simulink model "cube0_mpcpd"  (R2022b)
settings: Solver=VariableStepAuto  StartTime=0.0  StopTime=400  RelTol=1e-3  AbsTol=1e-3
undefined symbols (not defined in the file or in its folder): Angle, Axis
libraries: robotcorelib x2
settings Model: Creator=Abhijit  LastModifiedBy=abhij
settings SolverCC: AutoScaleAbsTol=off  AlgebraicLoopSolver=TrustRegion  MaxZcPerStep=1
settings DebuggingCC: UnconnectedInputMsg=warning  UnconnectedOutputMsg=warning  UnconnectedLineMsg=warning  SymbolicDimsDataTypeCodeGenerationDiagnostic=none  SFMachineParentedDataDiag=warning
settings ModelReferenceCC: EnableRefExpFcnMdlSchedulingChecks=on
settings SFSimCC: CustomCodeUndefinedFunction=UseInterfaceOnly
settings RTWCC: DLArmComputeVersion=19.05
settings SimscapeCC: SimscapeLogType=all  SimscapeLogSimulationStatistics=on  SimscapeLogDataHistory=10000

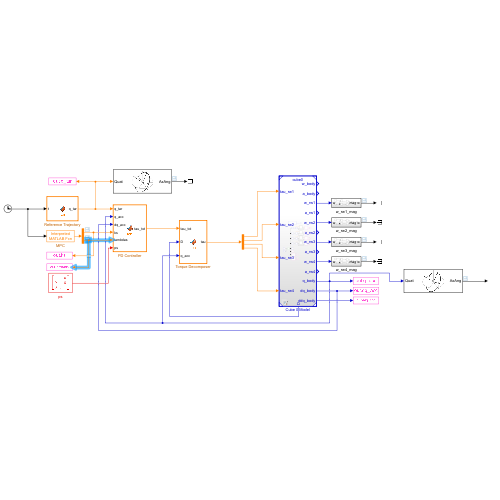
[thumbnail: Simulink's stored preview of the top-level diagram]
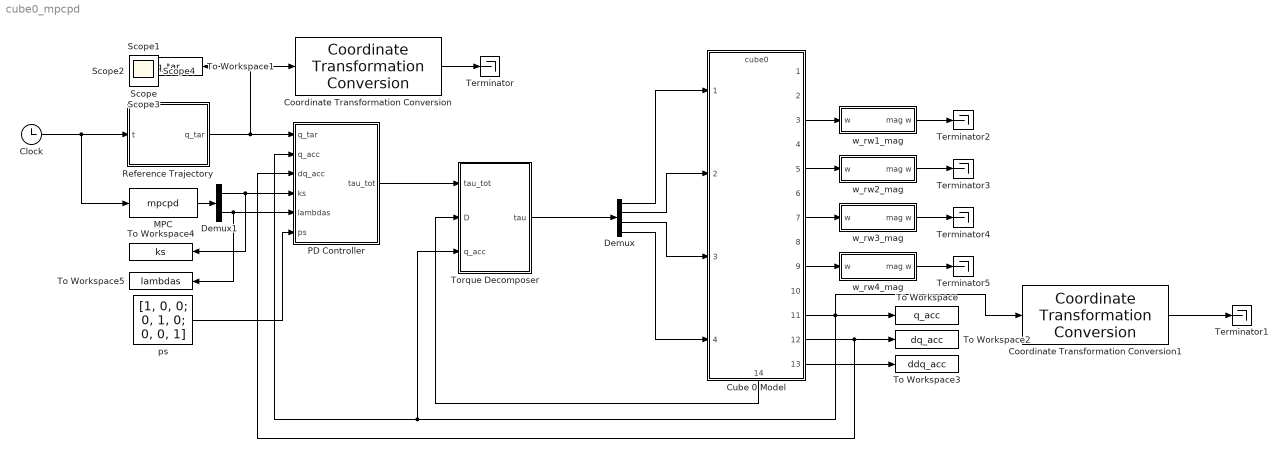
== system cube0_mpcpd ==
  Clock : Clock
  Coordinate Transformation Conversion : robotcorelib/Coordinate Transformation Conversion  InputRepresentation=Quaternion  InputEulerSequence=ZYX  ShowTrVecInputPort=on  OutputRepresentation=Axis-Angle  OutputEulerSequence=ZYX  ShowTrVecOutputPort=on  SimulateUsing=Interpreted execution
      settings: LibrarySourceBlock=navlib/Utilities/Coordinate Transformation Conversion
  Coordinate Transformation Conversion1 : robotcorelib/Coordinate Transformation Conversion  InputRepresentation=Quaternion  InputEulerSequence=ZYX  ShowTrVecInputPort=on  OutputRepresentation=Axis-Angle  OutputEulerSequence=ZYX  ShowTrVecOutputPort=on  SimulateUsing=Interpreted execution
      settings: LibrarySourceBlock=navlib/Utilities/Coordinate Transformation Conversion
  Cube 0 Model : ModelReference  ModelNameDialog=cube0.slx  SimulationMode=Normal  ModelReferenceVersion=1.24
      settings: PortSchema="{\"entries\":[{\"content\":{\"sides\":[{\"content\":{\"connectorIds\":[\"In1\",\"In2\",\"In3\",\"In4\"]},\"type\":\"ConnectorPlacement.EquallySpacedRectSide\",\"uuid\":\"36a9c944-f213-4c4e-b6f2-fa7d728627b0\"},{\"content\":{\"connectorIds\":[\"Out1\",\"Out2\",\"Out3\",\"Out4\",\"Out5\",\"Out6\",\"Out7\",\"Out8\",\"Out9\",\"Out10\",\"Out11\",\"Out12\",\"Out13\"],\"side\":\"RIGHT\"},\"type\":\"ConnectorPlacement.EquallySpacedRectSide\",\"uuid\":\"ad793041-f32f-405f-9966-9455be290c1c\"},{\"content\":{\"connectorIds\":[],\"side\":\"TOP\"},\"type\":\"ConnectorPlacement.EquallySpacedRectSide\",\"uuid\":\"a8d37d27-2c3a-480b-9200-d310321df053\"},{\"content\":{\"connectorIds\":[\"Out14\"],\"side\":\"BOTTOM\"},\"type\":\"ConnectorPlacement.EquallySpacedRectSide\",\"uuid\":\"42546c36-6810-4b9b-bafe-a7a09e10a567\"}]},\"type\":\"ConnectorPlacement.EquallySpacedConnector\",\"uuid\":\"5842ca05-faf4-4c84-934b-15246120a6a0\"}],\"packageUris\":[\"http://schema.mathworks.com/mf0/Connector/R2020b\"],\"version\":\"1.0\"}"
  Demux : Demux
  Demux1 : Demux  Outputs=2
  MPC : MATLABFcn  MATLABFcn=mpcpd  OutputDimensions=6
  PD Controller : MATLAB Function  TreatAsAtomicUnit=on
  Reference Trajectory : MATLAB Function  TreatAsAtomicUnit=on
  Terminator{,1..5} (6 alike) : Terminator
  To Workspace : ToWorkspace  VariableName=q_acc  SaveFormat=Timeseries  SampleTime=-1
  To Workspace1 : ToWorkspace  VariableName=q_tar  SaveFormat=Timeseries  SampleTime=-1
  To Workspace2 : ToWorkspace  VariableName=dq_acc  SaveFormat=Timeseries  SampleTime=-1
  To Workspace3 : ToWorkspace  VariableName=ddq_acc  SaveFormat=Timeseries  SampleTime=-1
  To Workspace4 : ToWorkspace  VariableName=ks  SaveFormat=Timeseries  SampleTime=-1
  To Workspace5 : ToWorkspace  VariableName=lambdas  SaveFormat=Timeseries  SampleTime=-1
  Torque Decomposer : MATLAB Function  TreatAsAtomicUnit=on
  ps : Constant  Value=[1, 0, 0; 0, 1, 0; 0, 0, 1]
  w_rw1_mag : Subsystem
  w_rw2_mag : Subsystem
  w_rw3_mag : Subsystem
  w_rw4_mag : Subsystem
  Scope{,1..4} (5 alike) : Scope
  wires:
  Clock/1 -> MPC/1, Reference Trajectory/1(t)
  Demux1/2 -> PD Controller/5(lambdas), To Workspace5/1
  Demux1/1 -> PD Controller/4(ks), To Workspace4/1
  ps/1 -> PD Controller/6(ps)
  Reference Trajectory/1(q_tar) -> Coordinate Transformation Conversion/1, To Workspace1/1, PD Controller/1(q_tar)
  MPC/1 -> Demux1/1
  Coordinate Transformation Conversion/1 -> Terminator/1
  w_rw3_mag/1(mag w) -> Terminator4/1
  Cube 0 Model/5 -> w_rw2_mag/1(w)
  w_rw1_mag/1(mag w) -> Terminator2/1
  Cube 0 Model/12 -> PD Controller/3(dq_acc), To Workspace2/1
  Cube 0 Model/9 -> w_rw4_mag/1(w)
  Demux/2 -> Cube 0 Model/2
  Cube 0 Model/7 -> w_rw3_mag/1(w)
  Cube 0 Model/3 -> w_rw1_mag/1(w)
  w_rw4_mag/1(mag w) -> Terminator5/1
  Demux/3 -> Cube 0 Model/3
  Cube 0 Model/13 -> To Workspace3/1
  Demux/4 -> Cube 0 Model/4
  Demux/1 -> Cube 0 Model/1
  Coordinate Transformation Conversion1/1 -> Terminator1/1
  Cube 0 Model/14 -> Torque Decomposer/2(D)
  w_rw2_mag/1(mag w) -> Terminator3/1
  Cube 0 Model/11 -> To Workspace/1, Coordinate Transformation Conversion1/1, PD Controller/2(q_acc), Torque Decomposer/3(q_acc)
  Torque Decomposer/1(tau) -> Demux/1
  PD Controller/1(tau_tot) -> Torque Decomposer/1(tau_tot)

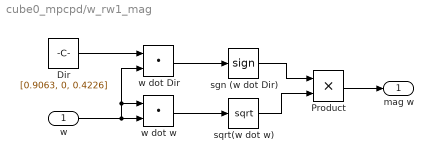
== system cube0_mpcpd/w_rw1_mag ==
  w : Inport
  Dir : Constant  Value=[0.9063, 0, 0.4226]
  Product : Product
  sgn (w dot Dir) : Signum
  sqrt(w dot w) : Sqrt
  w dot Dir : DotProduct  OutDataTypeStr=Inherit: Inherit via internal rule
  w dot w : DotProduct  OutDataTypeStr=Inherit: Inherit via internal rule
  mag w : Outport
  wires:
  w dot Dir/1 -> sgn (w dot Dir)/1
  w/1 -> w dot Dir/2, w dot w/1, w dot w/2
  w dot w/1 -> sqrt(w dot w)/1
  Product/1 -> mag w/1
  sqrt(w dot w)/1 -> Product/2
  Dir/1 -> w dot Dir/1
  sgn (w dot Dir)/1 -> Product/1

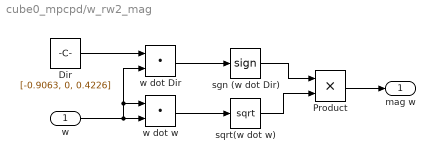
== system cube0_mpcpd/w_rw2_mag ==
  w : Inport
  Dir : Constant  Value=[-0.9063, 0, 0.4226]
  Product : Product
  sgn (w dot Dir) : Signum
  sqrt(w dot w) : Sqrt
  w dot Dir : DotProduct  OutDataTypeStr=Inherit: Inherit via internal rule
  w dot w : DotProduct  OutDataTypeStr=Inherit: Inherit via internal rule
  mag w : Outport
  wires:
  w/1 -> w dot Dir/2, w dot w/1, w dot w/2
  w dot w/1 -> sqrt(w dot w)/1
  Product/1 -> mag w/1
  sqrt(w dot w)/1 -> Product/2
  Dir/1 -> w dot Dir/1
  w dot Dir/1 -> sgn (w dot Dir)/1
  sgn (w dot Dir)/1 -> Product/1

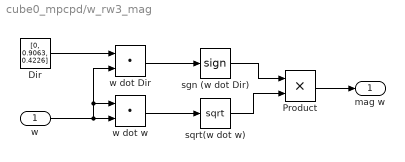
== system cube0_mpcpd/w_rw3_mag ==
  w : Inport
  Dir : Constant  Value=[0, 0.9063, 0.4226]
  Product : Product
  sgn (w dot Dir) : Signum
  sqrt(w dot w) : Sqrt
  w dot Dir : DotProduct  OutDataTypeStr=Inherit: Inherit via internal rule
  w dot w : DotProduct  OutDataTypeStr=Inherit: Inherit via internal rule
  mag w : Outport
  wires:
  w/1 -> w dot Dir/2, w dot w/1, w dot w/2
  w dot w/1 -> sqrt(w dot w)/1
  Product/1 -> mag w/1
  sqrt(w dot w)/1 -> Product/2
  Dir/1 -> w dot Dir/1
  w dot Dir/1 -> sgn (w dot Dir)/1
  sgn (w dot Dir)/1 -> Product/1

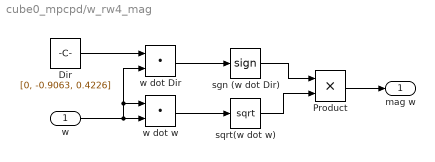
== system cube0_mpcpd/w_rw4_mag ==
  w : Inport
  Dir : Constant  Value=[0, -0.9063, 0.4226]
  Product : Product
  sgn (w dot Dir) : Signum
  sqrt(w dot w) : Sqrt
  w dot Dir : DotProduct  OutDataTypeStr=Inherit: Inherit via internal rule
  w dot w : DotProduct  OutDataTypeStr=Inherit: Inherit via internal rule
  mag w : Outport
  wires:
  w/1 -> w dot Dir/2, w dot w/1, w dot w/2
  w dot w/1 -> sqrt(w dot w)/1
  Product/1 -> mag w/1
  sqrt(w dot w)/1 -> Product/2
  Dir/1 -> w dot Dir/1
  w dot Dir/1 -> sgn (w dot Dir)/1
  sgn (w dot Dir)/1 -> Product/1

== matlab function cube0_mpcpd/PD Controller ==
  data: tau_tot output; q_tar input; q_acc input; dq_acc input; ks input; lambdas input; ps input
function tau_tot = fcn(q_tar, q_acc, dq_acc, ks, lambdas, ps)
    tau_tot = pdcontroller(q_tar, q_acc, dq_acc, ks, lambdas, ps);

== matlab function cube0_mpcpd/Reference Trajectory ==
  settings: updateMethod=CONTINUOUS
  data: t input; q_tar output
function q_tar = fcn(t)
     q_tar = refpath(t, 1);
end

== matlab function cube0_mpcpd/Torque Decomposer ==
  data: tau_tot input; tau output; D input; q_acc input
function tau = fcn(tau_tot, D, q_acc)
    tau = taudecomp(tau_tot, D, q_acc);
end
